simulink model "Commande_Profil_Position"  (R2024b)
settings: Solver=VariableStepAuto  StartTime=0.0  StopTime=1.3  RelTol=1e-3
undefined symbols (not defined in the file): amax, KD_EPOS, Kem, KI_EPOS, Kii_EPOS, Kip_EPOS, KP_EPOS, kr, M_axe, M_m, nm, r, rkr, Rm, t1, t2, t3, tr
libraries: fl_lib x23, nesl_utility x10, simulink x4
settings Model: Creator=xpess  LastModifiedBy=xpess
settings SolverCC: ZeroCrossAlgorithm=Adaptive
settings DebuggingCC: IgnoredZcDiagnostic=none
settings RTWCC: GPUComputeCapability=3.5

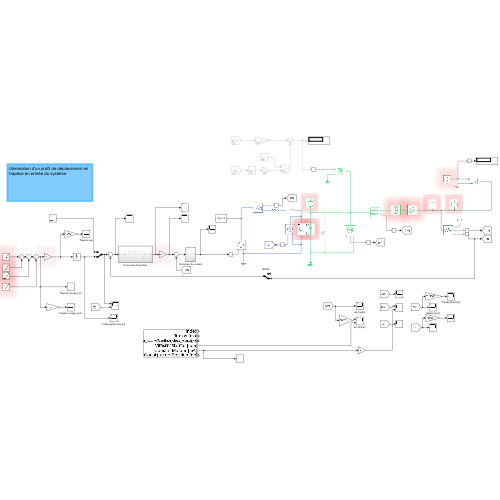
[thumbnail: Simulink's stored preview of the top-level diagram]
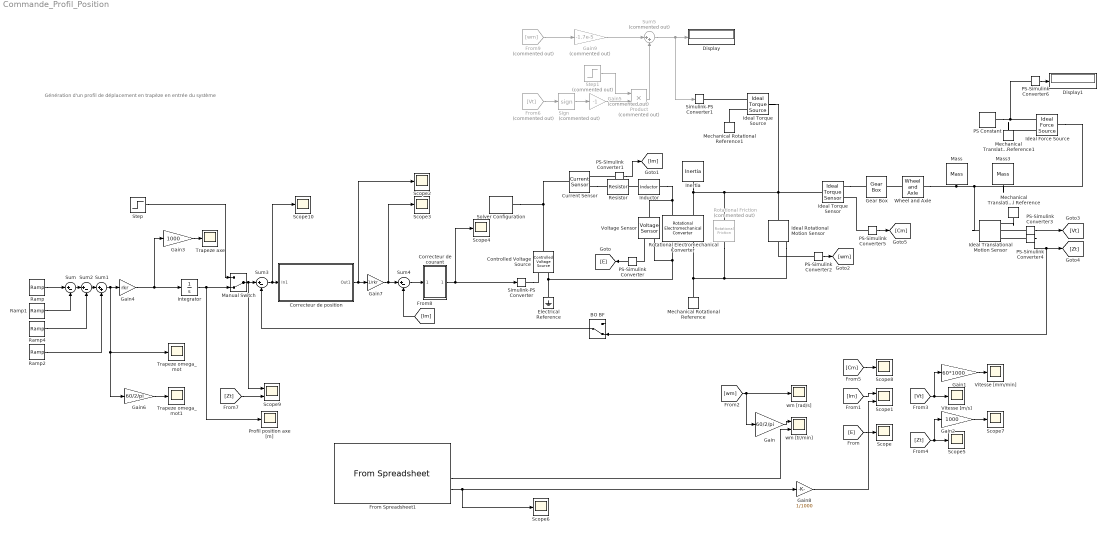
== system Commande_Profil_Position ==
  note: Génération d'un profil de déplacement en trapèze en entrée du système
  BO BF : ManualSwitch  CurrentSetting=0
  Controlled Voltage Source : fl_lib/Electrical/Electrical Sources/Controlled Voltage Source
  Correcteur de courant : Subsystem
  Correcteur de position : Subsystem
  Current Sensor : fl_lib/Electrical/Electrical Sensors/Current Sensor
  Display : Display
  Display1 : Display
  Electrical Reference : fl_lib/Electrical/Electrical Elements/Electrical Reference
  From Spreadsheet1 : FromSpreadsheet  FileName=C:\GitHub\TP_Corriges\04_Comax\Mesures\Profil_300mm_0m\Profil_Position_300mm_Matlab.xlsx  SheetName=Profil_Position_300mm
  From6 : From  Commented=on  GotoTag=Vt
  From9 : From  Commented=on  GotoTag=wm
  Gain : Gain  Gain=60/2/pi
  Gain1 : Gain  Gain=60*1000
  Gain2 : Gain  Gain=1000
  Gain3 : Gain  Gain=1000
  Gain4 : Gain  Gain=rkr
  Gain5 : Gain  Commented=on  Gain=-1
  Gain6 : Gain  Gain=60/2/pi
  Gain7 : Gain  Gain=1/rkr
  Gain8 : Gain  Gain=1/1000
  Gain9 : Gain  Commented=on  Gain=-1.7e-5
  Gear Box : fl_lib/Mechanical/Mechanisms/Gear Box  ratio=1/kr  t_in_specify=off  t_in_priority=None  t_in=0 N*m  t_in_nominal_specify=off  t_in_nominal_value=1  t_in_nominal_unit=N*m  t_out_specify=off  t_out_priority=None  t_out=0 N*m  t_out_nominal_specify=off  t_out_nominal_value=1  t_out_nominal_unit=N*m
  Ideal Force Source : fl_lib/Mechanical/Mechanical Sources/Ideal Force Source
  Ideal Rotational Motion Sensor : fl_lib/Mechanical/Mechanical Sensors/Ideal Rotational Motion Sensor  reference=foundation.enum.MeasurementReference.difference  acceleration_port=false  velocity_port=true  position_port=true  wrap_angle=false  offset=0 rad
  Ideal Torque Sensor : fl_lib/Mechanical/Mechanical Sensors/Ideal Torque Sensor
  Ideal Torque Source : fl_lib/Mechanical/Mechanical Sources/Ideal Torque Source
  Ideal Translational Motion Sensor : fl_lib/Mechanical/Mechanical Sensors/Ideal Translational Motion Sensor  reference=foundation.enum.MeasurementReference.difference  acceleration_port=false  velocity_port=true  position_port=true  offset=0 m
  Inductor : fl_lib/Electrical/Electrical Elements/Inductor  l=Lm H  r=0 Ohm  g=1e-9 1/Ohm  i_specify=off  i_priority=None  i=0 A  i_nominal_specify=off  i_nominal_value=1  i_nominal_unit=A  v_specify=off  v_priority=None  v=0 V  v_nominal_specify=off  v_nominal_value=1  v_nominal_unit=V  i_L_specify=off  i_L_priority=High  i_L=0 A  i_L_nominal_specify=off  i_L_nominal_value=1  i_L_nominal_unit=A
  Inertia : fl_lib/Mechanical/Rotational Elements/Inertia  inertia=J kg*m^2  num_ports=foundation.enum.numPorts2.one  w_specify=off  w_priority=High  w=0 rad/s  w_nominal_specify=off  w_nominal_value=1  w_nominal_unit=rad/s  t_specify=off  t_priority=None  t=0 N*m  t_nominal_specify=off  t_nominal_value=1  t_nominal_unit=N*m
  Integrator : Integrator
  Manual Switch : ManualSwitch  CurrentSetting=0
  Mass : fl_lib/Mechanical/Translational Elements/Mass  mass=M_axe kg  num_ports=foundation.enum.numPorts2.one  v_specify=off  v_priority=High  v=0 m/s  v_nominal_specify=off  v_nominal_value=1  v_nominal_unit=m/s  f_specify=off  f_priority=None  f=0 N  f_nominal_specify=off  f_nominal_value=1  f_nominal_unit=N
  Mass3 : fl_lib/Mechanical/Translational Elements/Mass  mass=M_m*nm kg  num_ports=foundation.enum.numPorts2.one  v_specify=off  v_priority=High  v=0 m/s  v_nominal_specify=off  v_nominal_value=1  v_nominal_unit=m/s  f_specify=off  f_priority=None  f=0 N  f_nominal_specify=off  f_nominal_value=1  f_nominal_unit=N
  Mechanical Rotational Reference : fl_lib/Mechanical/Rotational Elements/Mechanical Rotational Reference
  Mechanical Rotational Reference1 : fl_lib/Mechanical/Rotational Elements/Mechanical Rotational Reference
  Mechanical Translational Reference : fl_lib/Mechanical/Translational Elements/Mechanical Translational Reference
  Mechanical Translational Reference1 : fl_lib/Mechanical/Translational Elements/Mechanical Translational Reference
  PS Constant : fl_lib/Physical Signals/Sources/PS Constant  constant=-9.81*(M_axe+nm*M_m)
  PS-Simulink Converter{,1..6} (7 alike) : nesl_utility/PS-Simulink Converter  PhysicalDomain=network_engine_domain  SubClassName=ps_output  LeftPortType=input  RightPortType=output  PseudoPeriodic=off  Frequencies=[]  VectorFormat=inherit  Unit=inherit  AffineConversion=off
  Product : Product  Commented=on
  Profil position axe [m] : Scope
  Ramp : simulink/Sources/Ramp  slope=amax  start=tr  InitialOutput=0
  Ramp1 : simulink/Sources/Ramp  slope=amax  start=t1+tr  InitialOutput=0
  Ramp2 : simulink/Sources/Ramp  slope=amax  start=t3+tr  InitialOutput=0
  Ramp4 : simulink/Sources/Ramp  slope=amax  start=t2+tr  InitialOutput=0
  Resistor : fl_lib/Electrical/Electrical Elements/Resistor  R=Rm Ohm  i_specify=off  i_priority=None  i=0 A  i_nominal_specify=off  i_nominal_value=1  i_nominal_unit=A  v_specify=off  v_priority=None  v=0 V  v_nominal_specify=off  v_nominal_value=1  v_nominal_unit=V
  Rotational Electromechanical Converter : fl_lib/Electrical/Electrical Elements/Rotational Electromechanical Converter  K=Kem V/rpm  i_specify=off  i_priority=None  i=0 A  i_nominal_specify=off  i_nominal_value=1  i_nominal_unit=A  v_specify=off  v_priority=None  v=0 V  v_nominal_specify=off  v_nominal_value=1  v_nominal_unit=V  t_specify=off  t_priority=None  t=0 N*m  t_nominal_specify=off  t_nominal_value=1  t_nominal_unit=N*m  w_specify=off  w_priority=None  w=0 rad/s  w_nominal_specify=off  w_nominal_value=1  w_nominal_unit=rad/s
  Rotational Friction : fl_lib/Mechanical/Rotational Elements/Rotational Friction  Commented=on  brkwy_trq=0.024 N*m  brkwy_vel=1/10 rad/s  Col_trq=0.024 N*m  visc_coef=1.7e-5 N*m*s/rad  w_specify=off  w_priority=None  w=0 rad/s  w_nominal_specify=off  w_nominal_value=1  w_nominal_unit=rad/s  t_specify=off  t_priority=None  t=0 N*m  t_nominal_specify=off  t_nominal_value=1  t_nominal_unit=N*m
  Scope{,2..8,10} (9 alike) : Scope
  Scope1 : Scope  NumInputPorts=2
  Scope9 : Scope  NumInputPorts=2
  Sign : Signum  Commented=on
  Simulink-PS Converter : nesl_utility/Simulink-PS Converter  PhysicalDomain=network_engine_domain  SubClassName=ps_input  LeftPortType=input  RightPortType=output  PseudoPeriodic=off  Frequencies=[]  NoiseDistribution=none  NoiseParameters=[]  Unit=1  AffineConversion=off  FilteringAndDerivatives=provide  SimscapeFilterOrder=1  InputFilterTimeConstant=0.001  UdotUserProvided=0
  Simulink-PS Converter1 : nesl_utility/Simulink-PS Converter  PhysicalDomain=network_engine_domain  SubClassName=ps_input  LeftPortType=input  RightPortType=output  PseudoPeriodic=off  Frequencies=[]  NoiseDistribution=none  NoiseParameters=[]  Unit=1  AffineConversion=off  FilteringAndDerivatives=provide  SimscapeFilterOrder=1  InputFilterTimeConstant=0.001  UdotUserProvided=0
  Solver Configuration : nesl_utility/Solver Configuration  PhysicalDomain=network_engine_domain  SubClassName=solver  LeftPortType=input  RightPortType=generic  Tones=[]  Harmonics=[]  SimulateNoise=off  Profile=off  UseLocalSampling=off  EnableSwitchedLinearOptims=on  FrequencyDomain=off  UseCCode=off  RelTol=0.001  AbsTol=0.001  MinStep=1e-09  ToWorkspace=off  RevertToSquareIcSolve=off  NumHomotopyIterations=100  PhasorMode=off  PhasorModeNumHarmonics=1  ConsistencySolver=NEWTON_XTOL_AFTER_FTOL  IndexReductionMethod=DerivativeReplacement  DoDC=off  ResidualTolerance=1e-09  ConsistencyTolSource=GLOBAL  ConsistencyAbsTol=0.001  ConsistencyRelTol=0.001  ConsistencyTolFactor=0.001  UseLocalSolver=off  LocalSolverChoice=NE_BACKWARD_EULER_ADVANCER  ResolveIndetEquations=on  FunctionEvalNumThread=1  LocalSolverSampleTime=0.001  DoFixedCost=off  MaxNonlinIter=3  MaxModeIter=2  ComputeImpulses=off  ImpulseIterations=2  LinearAlgebra=auto  LinearAlgebraNumThread=0  EquationFormulation=NE_TIME_EF  DelaysMemoryBudget=1024  AutomaticFiltering=on  FilteringTimeConstant=0.001  PartitionStorageMethod=AS_NEEDED  PartitionMemoryBudget=1024  PartitionMethod=ROBUST  MultibodyUseLocalSolver=off  MultibodyLocalSolverChoice=ODE1  MultibodyLocalSolverSampleTime=0.001
  Step : Step  Time=.5  After=10  SampleTime=0
  Step1 : Step  Commented=on  Time=0  After=0.02  SampleTime=0
  Sum{,2..4} (4 alike) : Sum  Inputs=|+-
  Sum1 : Sum  Inputs=|++
  Sum5 : Sum  Commented=on  Inputs=|++
  Trapeze axe : Scope
  Trapeze omega_mot : Scope
  Trapeze omega_mot1 : Scope
  Vitesse [m/s] : Scope
  Vitesse [mm/min] : Scope
  Voltage Sensor : fl_lib/Electrical/Electrical Sensors/Voltage Sensor
  Wheel and Axle : fl_lib/Mechanical/Mechanisms/Wheel and Axle  R=r m  or=1  t_specify=off  t_priority=None  t=0 N*m  t_nominal_specify=off  t_nominal_value=1  t_nominal_unit=N*m  f_specify=off  f_priority=None  f=0 N  f_nominal_specify=off  f_nominal_value=1  f_nominal_unit=N
  wm [rad/s] : Scope
  wm [tr/min] : Scope  NumInputPorts=2
  wires:
  PS-Simulink Converter/1 -> [E]
  [E] -> Scope/1
  PS-Simulink Converter1/1 -> [Im]
  [Im] -> Scope1/1
  PS-Simulink Converter2/1 -> [wm]
  [wm] -> Gain/1, wm [rad/s]/1
  Gain/1 -> wm [tr/min]/1
  [Vt] -> Gain1/1, Vitesse [m/s]/1
  [Zt] -> Gain2/1, Scope5/1
  Gain1/1 -> Vitesse [mm/min]/1
  Gain2/1 -> Scope7/1
  PS-Simulink Converter5/1 -> [Cm]
  [Cm] -> Scope8/1
  Ramp1/1 -> Sum/2
  Ramp/1 -> Sum/1
  Ramp4/1 -> Sum2/2
  Sum2/1 -> Sum1/1
  Sum/1 -> Sum2/1
  Ramp2/1 -> Sum1/2
  PS-Simulink Converter3/1 -> [Vt]
  Step/1 -> Manual Switch/1
  Sum1/1 -> Trapeze omega_mot/1, Gain6/1, Gain4/1
  Manual Switch/1 -> Scope9/1, Sum3/1
  From6/1 -> Sign/1
  Sign/1 -> Gain5/1
  Step1/1 -> Product/1
  Gain5/1 -> Product/2
  Product/1 -> Sum5/2
  PS-Simulink Converter6/1 -> Display1/1
  Gain4/1 -> Integrator/1, Gain3/1
  PS-Simulink Converter4/1 -> BO BF/2, [Zt]
  [Zt] -> Scope9/2
  BO BF/1 -> Sum3/2
  Integrator/1 -> Profil position axe [m]/1, Manual Switch/2
  Sum3/1 -> Scope10/1, Correcteur de position/1(In1)
  Correcteur de position/1(Out1) -> Gain7/1, Scope2/1
  [Im] -> Sum4/2
  Gain7/1 -> Scope3/1, Sum4/1
  Sum4/1 -> Correcteur de courant/1(In1)
  Correcteur de courant/1(Out1) -> Scope4/1, Simulink-PS Converter/1
  Gain3/1 -> Trapeze axe/1
  Gain6/1 -> Trapeze omega_mot1/1
  From Spreadsheet1/5 -> Scope6/1, Gain8/1
  Gain8/1 -> Scope1/2
  From Spreadsheet1/4 -> wm [tr/min]/2
  From9/1 -> Gain9/1
  Gain9/1 -> Sum5/1
  Sum5/1 -> Display/1, Simulink-PS Converter1/1
  connections:
  Simulink-PS Converter/RConn1 -- Controlled Voltage Source/RConn1
  Solver Configuration/RConn1 -- Controlled Voltage Source/LConn1 -- Current Sensor/LConn1
  Inductor/LConn1 -- Resistor/RConn1
  Inductor/RConn1 -- Voltage Sensor/LConn1 -- Rotational Electromechanical Converter/LConn1
  Rotational Electromechanical Converter/RConn1 -- Voltage Sensor/RConn2 -- Electrical Reference/LConn1 -- Controlled Voltage Source/RConn2
  Mechanical Rotational Reference/LConn1 -- Rotational Electromechanical Converter/RConn2 -- Rotational Friction/RConn1 -- Ideal Rotational Motion Sensor/RConn1
  Inertia/LConn1 -- Ideal Torque Sensor/LConn1 -- Ideal Torque Source/LConn1 -- Ideal Rotational Motion Sensor/LConn1 -- Rotational Friction/LConn1 -- Rotational Electromechanical Converter/LConn2
  PS-Simulink Converter/LConn1 -- Voltage Sensor/RConn1
  Current Sensor/RConn2 -- Resistor/LConn1
  PS-Simulink Converter1/LConn1 -- Current Sensor/RConn1
  PS-Simulink Converter2/LConn1 -- Ideal Rotational Motion Sensor/RConn2
  Wheel and Axle/LConn1 -- Gear Box/RConn1
  Wheel and Axle/RConn1 -- Ideal Force Source/LConn1 -- Mass3/LConn1 -- Ideal Translational Motion Sensor/LConn1 -- Mass/LConn1
  Mechanical Translational Reference/LConn1 -- Ideal Translational Motion Sensor/RConn1
  PS-Simulink Converter3/LConn1 -- Ideal Translational Motion Sensor/RConn2
  PS-Simulink Converter4/LConn1 -- Ideal Translational Motion Sensor/RConn3
  Ideal Torque Sensor/RConn1 -- Gear Box/LConn1
  PS-Simulink Converter5/LConn1 -- Ideal Torque Sensor/RConn2
  Ideal Torque Source/RConn2 -- Mechanical Rotational Reference1/LConn1
  Ideal Torque Source/RConn1 -- Simulink-PS Converter1/RConn1
  PS Constant/RConn1 -- PS-Simulink Converter6/LConn1 -- Ideal Force Source/RConn1
  Mechanical Translational Reference1/LConn1 -- Ideal Force Source/RConn2

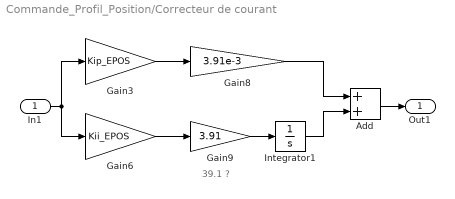
== system Commande_Profil_Position/Correcteur de courant ==
  note: 39.1 ?
  In1 : Inport
  Add : Sum
  Gain3 : Gain  Gain=Kip_EPOS
  Gain6 : Gain  Gain=Kii_EPOS
  Gain8 : Gain  Gain=3.91e-3
  Gain9 : Gain  Gain=3.91
  Integrator1 : Integrator
  Out1 : Outport
  wires:
  Gain9/1 -> Integrator1/1
  In1/1 -> Gain3/1, Gain6/1
  Add/1 -> Out1/1
  Integrator1/1 -> Add/2
  Gain6/1 -> Gain9/1
  Gain8/1 -> Add/1
  Gain3/1 -> Gain8/1

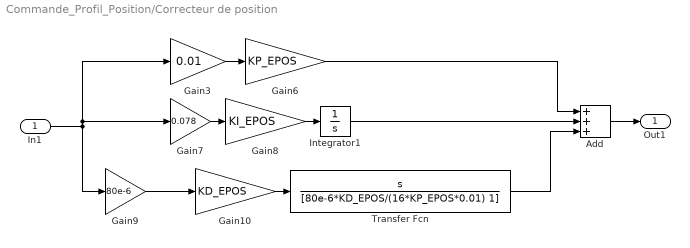
== system Commande_Profil_Position/Correcteur de position ==
  In1 : Inport
  Add : Sum  Inputs=+++
  Gain10 : Gain  Gain=KD_EPOS
  Gain3 : Gain  Gain=0.01
  Gain6 : Gain  Gain=KP_EPOS
  Gain7 : Gain  Gain=0.078
  Gain8 : Gain  Gain=KI_EPOS
  Gain9 : Gain  Gain=80e-6
  Integrator1 : Integrator
  Transfer Fcn : TransferFcn  Numerator=[1 0]  Denominator=[80e-6*KD_EPOS/(16*KP_EPOS*0.01) 1]
  Out1 : Outport
  wires:
  Gain8/1 -> Integrator1/1
  Transfer Fcn/1 -> Add/3
  Gain10/1 -> Transfer Fcn/1
  Add/1 -> Out1/1
  Gain3/1 -> Gain6/1
  Integrator1/1 -> Add/2
  In1/1 -> Gain7/1, Gain3/1, Gain9/1
  Gain6/1 -> Add/1
  Gain7/1 -> Gain8/1
  Gain9/1 -> Gain10/1
